simulink model "ejercicio1c"  (R2015a)
settings: Solver=ode45  StartTime=0.0  StopTime=4  RelTol=1e-3
settings Model: CovModelRefEnable=off  Creator=xmax1946  LastModifiedBy=xmax1946
settings DataIOCC: SaveFormat=Dataset
settings HardwareCC: ProdBitPerPointer=64  ProdLargestAtomicFloat=Float  ProdIntDivRoundTo=Zero  ProdEndianess=LittleEndian  ProdHWDeviceType=Specified
settings GRTTargetCC: GeneratePreprocessorConditionals=Use local settings

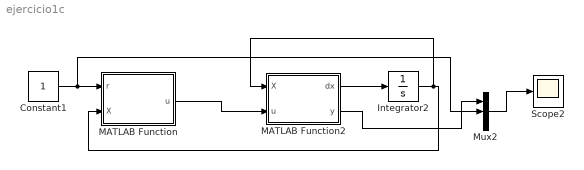
== system ejercicio1c ==
  Constant1 : Constant
  Integrator2 : Integrator  InitialCondition=[0;0;0;0;0;0]
  MATLAB Function : MATLAB Function  TreatAsAtomicUnit=on
      settings: PermitHierarchicalResolution=ParametersOnly
  MATLAB Function2 : MATLAB Function  TreatAsAtomicUnit=on
      settings: PermitHierarchicalResolution=ParametersOnly
  Mux2 : Mux  Inputs=3
  Scope2 : Scope
      settings: TimeRange=auto  MaxDataPoints=5000  SaveToWorkspace=off  YMin=-2.08336  YMax=8.75024  SampleTime=-1
  wires:
  Constant1/1 -> Mux2/2, MATLAB Function/1(r)
  MATLAB Function2/1(dx) -> Integrator2/1
  Integrator2/1 -> MATLAB Function2/1(X), MATLAB Function/2(X)
  MATLAB Function/1(u) -> MATLAB Function2/2(u)
  MATLAB Function2/2(y) -> Mux2/1
  Mux2/1 -> Scope2/1

== matlab function ejercicio1c/MATLAB Function ==
  data: u output; r input; X input
function u = fcn(r,X)
K=[-.566,.001,1.038,.1254,1.76,.596]*1e+02;
K=[-.359,.01,1.245,.125,1.1395,.389]*1e+02;
u=K(5)*r-K*X;

== matlab function ejercicio1c/MATLAB Function2 ==
  data: X input; dx output; u input; y output
function [dx,y] = fcn(X,u)
m1=2;
m2=1;
m3=1;
v1=1;
v2=1;
v3=1;
v4=1;
v5=1;
k=2;
A=[0,1,0,0,0,0;
  -k/m1,(-v2-v4-v1)/m1,k/m1,v2/m1,0,v4/m1
  0,0,0,1,0,0 
  k/m2,v2/m2,-k/m2,(-v2-v5)/m2,0,v5/m2
  0,0,0,0,0,1
  0,v4/m3,0,v5/m3,0,(-v4-v3-v5)/m3
    ];
B=[0;0;0;1/m2;0;0];
C=[0,0,0,0,1,0];

dx=A*X+B*u;
y = C*X;
